simulink model "model_kalman_190510"  (R2016b)
settings: Solver=VariableStepAuto  StartTime=0.0  StopTime=t_sim  RelTol=1e-3
values from neighbouring files (symbols this model uses):
  A = [1 Ts; 0 1]    [kalman_190510.m]    (also in objfunc.m)
  B = [0;0]    [kalman_190510.m]    (also in objfunc.m)
  C = [1 0; 0 1]    [kalman_190510.m]    (also in objfunc.m)
  D = [0;0]    [kalman_190510.m]    (also in objfunc.m)
  noise_hall = 0.01    [kalman_190510.m]    (also in objfunc.m)
  noise_pos_meas = 0.51    [kalman_190510.m]    (also in objfunc.m)
  R = [noise_pos_meas 0; 0 noise_hall]    [kalman_190510.m]    (also in objfunc.m)
  Ts = 0.1    [kalman_190510.m]    (also in objfunc.m)
undefined symbols (not defined in the file or in its folder): DiscIntNeverNeededParam, Discrete, Time
libraries: ctrlSharedLib x1, simulink x1
settings Model: Creator=Cécile  LastModifiedBy=maximefeingesicht
settings SFSimCC: SimUseLocalCustomCode=on
settings RTWCC: RTWUseLocalCustomCode=on

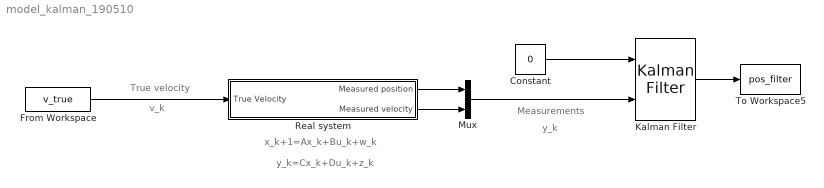
== system model_kalman_190510 ==
  note: y_k=Cx_k+Du_k+z_k
  note: x_k+1=Ax_k+Bu_k+w_k
  note: y_k
  note: v_k
  note: Measurements
  note: True velocity
  Constant : Constant  Value=0  SampleTime=-1
  From Workspace : FromWorkspace  VariableName=v_true  SampleTime=Ts  Interpolate=off  OutputAfterFinalValue=Holding final value
  "Kalman Filter " : ctrlSharedLib/Kalman Filter  TimeDomain=Discrete-Time  UseCurrentEstimator=on  ModelSource=Individual A, B, C, D matrices  ModelSourceVariable=ss(0.95,1,1,0,1)  A=A  B=B  C=C  D=D  NumberOfStates=1  NumberOfInputs=1  NumberOfOutputs=1  InitialEstimateSource=Dialog  X0=0  P0=10  UseK=off  UseGH=off  NumberOfProcessNoiseInputs=1  G=1  TimeInvariantG=on  H=0  TimeInvariantH=on  Q=Q  TimeInvariantQ=on  R=R  TimeInvariantR=on  N=0  TimeInvariantN=on  AddInputPort=on  AddEnablePort=off  OutputEstimatedY=off  OutputP=off  Ts=-1
  Mux : Mux  Inputs=2
  Real system : Subsystem
  To Workspace5 : ToWorkspace  VariableName=pos_filter  SaveFormat=Timeseries  SampleTime=-1
  wires:
  "Kalman Filter "/1 -> To Workspace5/1
  Mux/1 -> "Kalman Filter "/2
  From Workspace/1 -> Real system/1(True Velocity)
  Real system/1(Measured position) -> Mux/1
  Real system/2(Measured velocity) -> Mux/2
  Constant/1 -> "Kalman Filter "/1

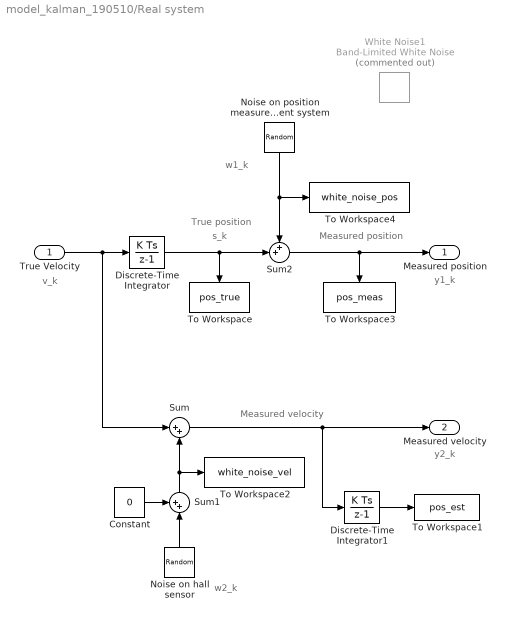
== system model_kalman_190510/Real system ==
  note: y2_k
  note: y1_k
  note: w2_k
  note: w1_k
  note: s_k
  note: v_k
  note: Measured position
  note: True position
  note: Measured velocity
  True Velocity : Inport
  " White Noise1" : simulink/Sources/Band-Limited White Noise  Commented=on  Cov=[0.2]  Ts=Ts  seed=rand()*25536
  Constant : Constant  Value=0
  Discrete-Time Integrator : DiscreteIntegrator  InitialConditionSetting=State (most efficient)  SampleTime=-1  ICPrevOutput=DiscIntNeverNeededParam  ICPrevScaledInput=DiscIntNeverNeededParam
  Discrete-Time Integrator1 : DiscreteIntegrator  InitialConditionSetting=State (most efficient)  SampleTime=-1  ICPrevOutput=DiscIntNeverNeededParam  ICPrevScaledInput=DiscIntNeverNeededParam
  Noise on hall sensor : RandomNumber  Variance=noise_hall  SampleTime=Ts
  Noise on position measurement system : RandomNumber  Variance=noise_pos_meas  SampleTime=Ts
  Sum : Sum  Inputs=|++
  Sum1 : Sum  Inputs=++|
  Sum2 : Sum  Inputs=++|
  To Workspace : ToWorkspace  VariableName=pos_true  SaveFormat=Timeseries  SampleTime=-1
  To Workspace1 : ToWorkspace  VariableName=pos_est  SaveFormat=Timeseries  SampleTime=-1
  To Workspace2 : ToWorkspace  VariableName=white_noise_vel  SaveFormat=Timeseries  SampleTime=-1
  To Workspace3 : ToWorkspace  VariableName=pos_meas  SaveFormat=Timeseries  SampleTime=-1
  To Workspace4 : ToWorkspace  VariableName=white_noise_pos  SaveFormat=Timeseries  SampleTime=-1
  Measured position : Outport
  Measured velocity : Outport  Port=2
  wires:
  Sum2/1 -> To Workspace3/1, Measured position/1
  Discrete-Time Integrator/1 -> Sum2/2, To Workspace/1
  True Velocity/1 -> Sum/1, Discrete-Time Integrator/1
  Sum1/1 -> Sum/2, To Workspace2/1
  Constant/1 -> Sum1/1
  Sum/1 -> Measured velocity/1, Discrete-Time Integrator1/1
  Noise on hall sensor/1 -> Sum1/2
  Discrete-Time Integrator1/1 -> To Workspace1/1
  Noise on position measurement system/1 -> To Workspace4/1, Sum2/1
